simulink model "linear_bonus_model"  (R2021b)
settings: Solver=VariableStepAuto  StartTime=0.0  StopTime=10.0  RelTol=1e-3
values from neighbouring files (symbols this model uses):
  AmpDen = [1 655.7 5.52e6]    [draft_model_variables.m]    (also in linear_model_variables.m = [1 655.7 7.704e5])
  AmpNum = [2.149e7]    [draft_model_variables.m]    (also in linear_model_variables.m = [3e06])
  B = 7e-4    (= 0.0007)    [draft_model_variables.m]    (also in linear_model_variables.m)
  CF = 1000    [derivative_filter.m]    (also in draft_model_variables.m = 1163; linear_model_variables.m = 10000)
  J1 = 2.60    (= 2.6)    [linear_model_variables.m]
  J2 = Jrot/1000 + 0.09    (= 0.0900831)    [linear_model_variables.m]
  K1 = 0.589    [draft_model_variables.m]
  K2 = 0.0753    [draft_model_variables.m]
  Kd1 = 109.6356    [draft_model_variables.m]    (also in linear_model_variables.m = 3)
  Kd2 = 99.9905    [draft_model_variables.m]    (also in linear_model_variables.m = 2)
  Ki1 = 1    [draft_model_variables.m]    (also in linear_model_variables.m = 0)
  Ki2 = 1    [draft_model_variables.m]    (also in linear_model_variables.m = 0)
  Kp1 = 20.9419    [draft_model_variables.m]    (also in linear_model_variables.m = 2)
  Kp2 = 19.9995    [draft_model_variables.m]    (also in linear_model_variables.m = 1)
  N = 10    [derivative_filter.m]    (also in draft_model_variables.m = 100)
  s = tf('s')    [draft_model_variables.m]
undefined symbols (not defined in the file or in its folder): gear1, gear2, gear3, J3, K3, ka1, ka2, ka3, Kd3, Ki3, km1, km2, km3, Kp3, L1, L2, L3, R1, R2, R3
libraries: cstblocks x3, simulink x3
settings Model: Creator=ncamp  LastModifiedBy=ncamp

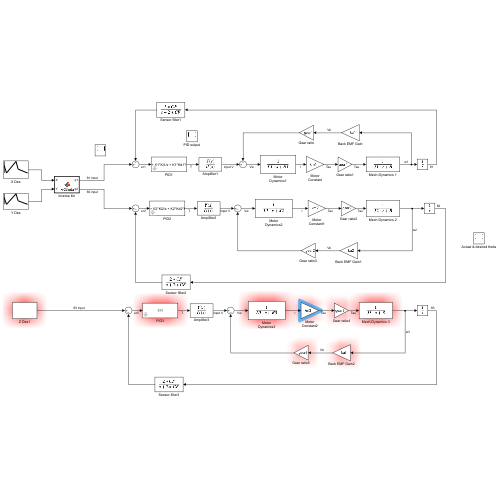
[thumbnail: Simulink's stored preview of the top-level diagram]
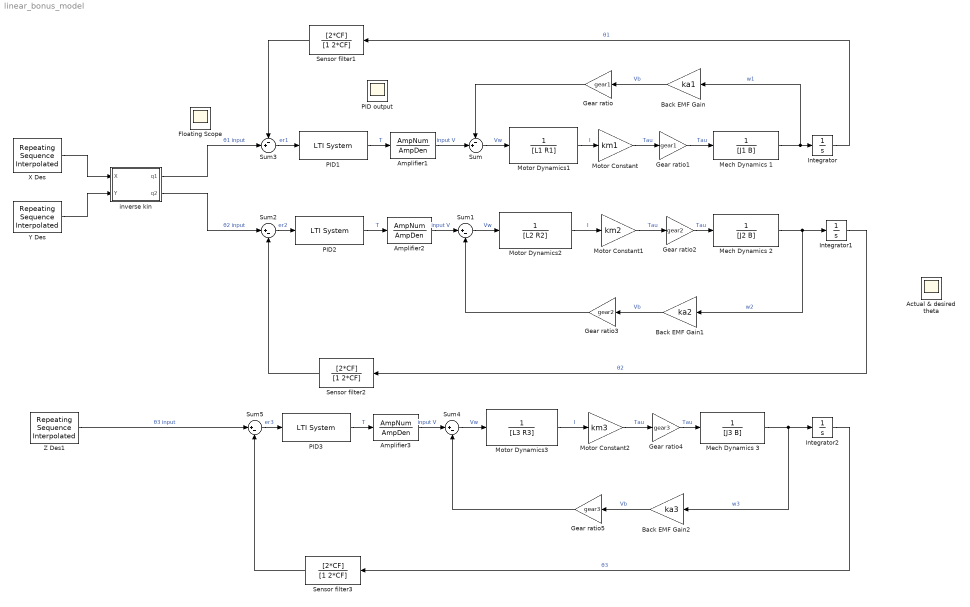
== system linear_bonus_model ==
  Actual & desired theta : Scope
      settings: Floating=on
  Amplifier1 : TransferFcn  Numerator=AmpNum  Denominator=AmpDen
  Amplifier2 : TransferFcn  Numerator=AmpNum  Denominator=AmpDen
  Amplifier3 : TransferFcn  Numerator=AmpNum  Denominator=AmpDen
  Back EMF Gain : Gain  Gain=ka1
  Back EMF Gain1 : Gain  Gain=ka2
  Back EMF Gain2 : Gain  Gain=ka3
  Floating Scope : Scope
      settings: Floating=on
  Gear ratio : Gain  Gain=gear1
  Gear ratio1 : Gain  Gain=gear1
  Gear ratio2 : Gain  Gain=gear2
  Gear ratio3 : Gain  Gain=gear2
  Gear ratio4 : Gain  Gain=gear3
  Gear ratio5 : Gain  Gain=gear3
  Integrator : Integrator
  Integrator1 : Integrator
  Integrator2 : Integrator
  Mech Dynamics 1 : TransferFcn  Denominator=[J1 B]
  Mech Dynamics 2 : TransferFcn  Denominator=[J2 B]
  Mech Dynamics 3 : TransferFcn  Denominator=[J3 B]
  Motor Constant : Gain  Gain=km1
  Motor Constant1 : Gain  Gain=km2
  Motor Constant2 : Gain  Gain=km3
  Motor Dynamics1 : TransferFcn  Denominator=[L1 R1]
  Motor Dynamics2 : TransferFcn  Denominator=[L2 R2]
  Motor Dynamics3 : TransferFcn  Denominator=[L3 R3]
  PID output : Scope
      settings: Floating=on
  PID1 : cstblocks/LTI System  sys=tf(K1*Kp1 + K1*Ki1/s + K1*Kd1*N*s/(s+N))  IC=[]
  PID2 : cstblocks/LTI System  sys=tf(K2*Kp2 + K2*Ki2/s + K2*Kd2*N*s/(s+N))  IC=[]
  PID3 : cstblocks/LTI System  sys=tf(K3*Kp3 + K3*Ki3/s + K3*Kd3*N*s/(s+N))  IC=[]
  Sensor filter1 : TransferFcn  Numerator=[2*CF]  Denominator=[1 2*CF]
  Sensor filter2 : TransferFcn  Numerator=[2*CF]  Denominator=[1 2*CF]
  Sensor filter3 : TransferFcn  Numerator=[2*CF]  Denominator=[1 2*CF]
  Sum : Sum  Inputs=-+|
  Sum{1..2,4..5} (4 alike) : Sum  Inputs=|+-
  Sum3 : Sum  Inputs=-+|
  X Des : simulink/Sources/Repeating Sequence Interpolated  OutValues=X  TimeValues=time  LookUpMeth=Interpolation-Use End Values  tsamp=0.001  OutMin=[]  OutMax=[]  OutDataTypeStr=double  OutputDataTypeScalingMode=double  OutDataType=fixdt(0,8)  OutScaling=2^-10
  Y Des : simulink/Sources/Repeating Sequence Interpolated  OutValues=Y  TimeValues=time  LookUpMeth=Interpolation-Use End Values  tsamp=0.001  OutMin=[]  OutMax=[]  OutDataTypeStr=double  OutputDataTypeScalingMode=double  OutDataType=fixdt(0,8)  OutScaling=2^-10
  Z Des1 : simulink/Sources/Repeating Sequence Interpolated  OutValues=Z  TimeValues=time  LookUpMeth=Interpolation-Use End Values  tsamp=0.001  OutMin=[]  OutMax=[]  OutDataTypeStr=double  OutputDataTypeScalingMode=double  OutDataType=fixdt(0,8)  OutScaling=2^-10
  inverse kin : MATLAB Function  TreatAsAtomicUnit=on
  wires:
  Gear ratio/1 -> Sum/1
  Sensor filter2/1 -> Sum2/2
  Sum1/1 -> Motor Dynamics2/1  "Vw"
  Mech Dynamics 1/1 -> Integrator/1, Back EMF Gain/1  "w1"
  inverse kin/2(q2) -> Sum2/1  "θ2 input"
  Mech Dynamics 2/1 -> Integrator1/1, Back EMF Gain1/1  "w2"
  Motor Dynamics2/1 -> Motor Constant1/1  "I"
  Sum/1 -> Motor Dynamics1/1  "Vw"
  Amplifier2/1 -> Sum1/1  "input V"
  Motor Constant/1 -> Gear ratio1/1  "Tau"
  Sum2/1 -> PID2/1  "er2"
  Back EMF Gain1/1 -> Gear ratio3/1  "Vb"
  Gear ratio1/1 -> Mech Dynamics 1/1  "Tau"
  Integrator/1 -> Sensor filter1/1  "θ1"
  Integrator1/1 -> Sensor filter2/1  "θ2"
  X Des/1 -> inverse kin/1(X)
  Motor Constant1/1 -> Gear ratio2/1  "Tau"
  Back EMF Gain/1 -> Gear ratio/1  "Vb"
  PID1/1 -> Amplifier1/1  "T"
  PID2/1 -> Amplifier2/1  "T"
  Sensor filter1/1 -> Sum3/1
  Y Des/1 -> inverse kin/2(Y)
  Amplifier1/1 -> Sum/2  "input V"
  Motor Dynamics1/1 -> Motor Constant/1  "I"
  Gear ratio2/1 -> Mech Dynamics 2/1  "Tau"
  inverse kin/1(q1) -> Sum3/2  "θ1 input"
  Sum3/1 -> PID1/1  "er1"
  Gear ratio3/1 -> Sum1/2
  Gear ratio5/1 -> Sum4/2
  Sum4/1 -> Motor Dynamics3/1  "Vw"
  Sensor filter3/1 -> Sum5/2
  PID3/1 -> Amplifier3/1  "T"
  Motor Constant2/1 -> Gear ratio4/1  "Tau"
  Integrator2/1 -> Sensor filter3/1  "θ3"
  Sum5/1 -> PID3/1  "er3"
  Amplifier3/1 -> Sum4/1  "input V"
  Motor Dynamics3/1 -> Motor Constant2/1  "I"
  Mech Dynamics 3/1 -> Integrator2/1, Back EMF Gain2/1  "w3"
  Gear ratio4/1 -> Mech Dynamics 3/1  "Tau"
  Back EMF Gain2/1 -> Gear ratio5/1  "Vb"
  Z Des1/1 -> Sum5/1  "θ3 input"

== matlab function linear_bonus_model/inverse kin ==
  data: X input; q1 output; Y input; q2 output
function [q1,q2] = xy2theta(X,Y)

% Inputs X,Y should be in mm
% Outputs q1, q2 are in rads

L1 = 275;   % Arm 1 length (mm)
L2 = 275;   % Arm 2 length (mm)

% Elbow down position
q1 = 2*atan((2*L1*Y - (- L1^4 + 2*L1^2*L2^2 + 2*L1^2*X^2 + 2*L1^2*Y^2 - L2^4 + 2*L2^2*X^2 + 2*L2^2*Y^2 - X^4 - 2*X^2*Y^2 - Y^4)^(1/2))/(L1^2 + 2*L1*X - L2^2 + X^2 + Y^2));
q2 =  2*atan(((- L1^2 + 2*L1*L2 - L2^2 + X^2 + Y^2)*(L1^2 + 2*L1*L2 + L2^2 - X^2 - Y^2))^(1/2)/(- L1^2 + 2*L1*L2 - L2^2 + X^2 + Y^2));


end
